simulink model "EVSimulation"  (R2020b)
settings: Solver=VariableStepAuto  StartTime=0.0  StopTime=600  FixedStep=0.5  RelTol=1e-3
model workspace (MAT data in the model file):
  AccessoryLoad = 0
  Af = 1.8
  C0 = 0.02
  Cd = 0.48
  airDensity = 1.225
  beta = 0
  energyCapacity = 30
  g = 9.81
  gearboxEfficiency = 90
  internalResistance = 0.05
  m = 840
  maxBrakeForce = 2000
  motorEfficiency = 90
  motorMaxPower = 40000
  motorMaxTorque = 83
  openCircuitVoltage = 140
  regenFraction = 1
  wheelRadius = 0.29
  windVel = 0
libraries: simulink x2, autolibshared x1, pid_lib x1
settings Model: SimulationMode=accelerator  OrderedModelArguments=off  Creator=Caleb  LastModifiedBy=Caleb

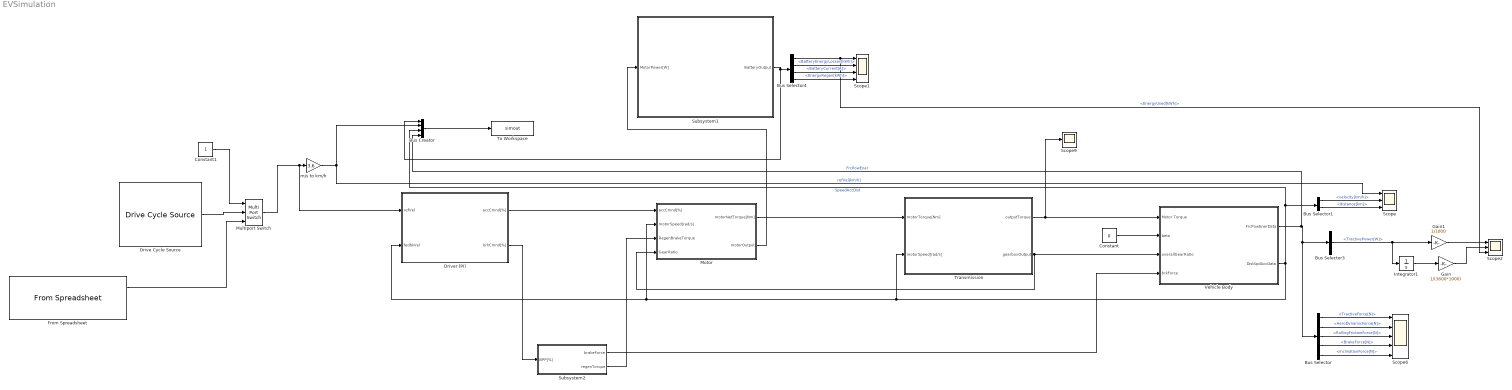
== system EVSimulation ==
  Bus Creator : BusCreator  Inputs=4
  Bus Selector : BusSelector  OutputSignals=TractiveForce[N],AeroDynamicForce[N],RollingFrictionForce[N],BrakeForce[N],InclinationForce[N]
  Bus Selector1 : BusSelector  OutputSignals=velocity[km/h],distance[km]
  Bus Selector3 : BusSelector  OutputSignals=TractivePower[W]
  Bus Selector4 : BusSelector  OutputSignals=EnergyUsed[kWh],BatteryEnergyLosses[kWh],BatteryCurrent[A],EnergyRegen[kWh]
  Constant : Constant  Value=0
  Constant1 : Constant
  Drive Cycle Source : autolibshared/Drive Cycle Source  cycleVar=US06  fileVar=cycleFTP75.mat  tfinal="600  seconds, Cyclic"  cycleRepeat=on  outAccPort=off  outGearPort=off  gearList=No gear data  t_wot1=5  xdot_woto=0  xdot_wot1=30  t_wot2=20  xdot_wot2=0  t_wotend=30  srcUnit=m/s  outUnit=m/s  srcAccUnit=m/s/s  outAccUnit=m/s^2  dt=0  aMode=1  faultOption=off  velBnd=2  velBndUnit=mph  inUnit=m/s  timeBnd=1  failOption=off  stopSim=off  maxFaultCnt=10  maxFaultTime=2  maxTotFaultTime=15  traceOption=off  dtTrace=1  traceWindow=10  lastDCname=FTP75 Velocity  lastOutUnit=mph  lastDT=0  lastTB=1  lastSB=2  forceCalcBound=off
      settings: SourceProductBaseCode=PW,MT,UV,VE,VP
  Driver (PI) : Subsystem
  From Spreadsheet : FromSpreadsheet  FileName=SpeedInputDrivecyle.xlsx  SheetName=Sheet2  ExtrapolationAfterLastDataPoint=Hold last value
  Gain : Gain  Gain=1/(3600*1000)
  Gain1 : Gain  Gain=1/1000
  Integrator1 : Integrator
  Motor : Subsystem
  Multiport Switch : MultiPortSwitch  Inputs=2
  Scope : Scope  NumInputPorts=3
  Scope1 : Scope  NumInputPorts=4
  Scope2 : Scope  NumInputPorts=3
  Scope6 : Scope  NumInputPorts=5
  Scope9 : Scope
  Subsystem1 : Subsystem
  Subsystem2 : Subsystem
  To Workspace : ToWorkspace  VariableName=simout  SaveFormat=Timeseries  SampleTime=-1
  Transmission : Subsystem
  Vehicle Body : Subsystem
  m/s to km/h : Gain  Gain=3.6
  wires:
  Motor/1(motorNetTorque[Nm]) -> Transmission/1(motorTorque[Nm])
  Transmission/1(outputTorque) -> Scope9/1, Vehicle Body/1(Motor Torque)
  Transmission/2(gearboxOutput) -> Motor/4(GearRatio), Vehicle Body/3(overallGearRatio)
  m/s to km/h/1 -> Bus Creator/2, Scope/1  "refVel[km/h]"
  Vehicle Body/1(FrcPowEnerData) -> Bus Creator/4, Bus Selector/1, Bus Selector3/1  "FrcPowEner"
  Vehicle Body/2(DistSpdAccData) -> Transmission/2(motorSpeed[rad/s]), Motor/2(motorSpeed[rad/s]), Driver (PI)/2(fedbkVel), Bus Creator/3, Bus Selector1/1  "SpeedAccDist"
  Bus Selector1/1 -> Scope/2  "<velocity[km/h]>"
  Bus Selector/5 -> Scope6/5  "<InclinationForce[N]>"
  Bus Selector3/1 -> Integrator1/1, Gain1/1  "<TractivePower[W]>"
  Subsystem1/1(BatteryOutput) -> Bus Creator/1, Bus Selector4/1
  Bus Selector4/1 -> Scope2/3, Scope1/1  "<EnergyUsed[kWh]>"
  Drive Cycle Source/1 -> Multiport Switch/2
  Bus Selector1/2 -> Scope/3  "<distance[km]>"
  Multiport Switch/1 -> Driver (PI)/1(refVel), m/s to km/h/1
  From Spreadsheet/1 -> Multiport Switch/3
  Constant1/1 -> Multiport Switch/1
  Integrator1/1 -> Gain/1
  Gain/1 -> Scope2/2
  Motor/2(motorOutput) -> Subsystem1/1(MotorPower[W])
  Bus Selector4/2 -> Scope1/2  "<BatteryEnergyLosses[kWh]>"
  Bus Selector4/3 -> Scope1/3  "<BatteryCurrent[A]>"
  Bus Creator/1 -> To Workspace/1
  Bus Selector/1 -> Scope6/1  "<TractiveForce[N]>"
  Driver (PI)/1(accCmnd[%]) -> Motor/1(accCmnd[%])
  Driver (PI)/2(brkCmnd[%]) -> Subsystem2/1(BPP[%])
  Gain1/1 -> Scope2/1
  Bus Selector/2 -> Scope6/2  "<AeroDynamicForce[N]>"
  Bus Selector/3 -> Scope6/3  "<RollingFrictionForce[N]>"
  Bus Selector/4 -> Scope6/4  "<BrakeForce[N]>"
  Constant/1 -> Vehicle Body/2(beta)
  Subsystem2/1(brakeForce) -> Vehicle Body/4(brkForce)
  Subsystem2/2(regenTorque) -> Motor/3(RegenBrakeTorque)
  Bus Selector4/4 -> Scope1/4  "<EnergyRegen[kWh]>"

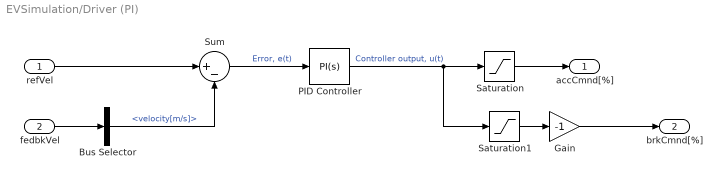
== system EVSimulation/Driver (PI) ==
  refVel : Inport
  fedbkVel : Inport  Port=2
  Bus Selector : BusSelector  OutputSignals=velocity[m/s]
  Gain : Gain  Gain=-1
  PID Controller : pid_lib/PID Controller  Controller=PI  Form=Parallel  TimeDomain=Continuous-time  UseExternalTs=off  SampleTime=-1  IntegratorMethod=Forward Euler  FilterMethod=Forward Euler  ControllerParametersSource=internal  P=200  I=1  D=0  UseFilter=on  N=1  TunerSelectOption=Transfer Function Based (PID Tuner App)  InitialConditionSource=internal  InitialConditionForIntegrator=0  InitialConditionForFilter=0  DifferentiatorICPrevScaledInput=0  ExternalReset=none  TrackingMode=off  Kt=1  LimitOutput=off  SatLimitsSource=internal  UpperSaturationLimit=inf  LowerSaturationLimit=-inf  LinearizeAsGain=on  AntiWindupMode=clamping  Kb=1  POutMin=[]  POutMax=[]  IOutMin=[]  IOutMax=[]  DOutMin=[]  DOutMax=[]  NOutMin=[]  NOutMax=[]  SumOutMin=[]  SumOutMax=[]  SaturationOutMin=[]  SaturationOutMax=[]  PParamMin=[]  PParamMax=[]  IParamMin=[]  IParamMax=[]  DParamMin=[]  DParamMax=[]  NParamMin=[]  NParamMax=[]  KbParamMin=[]  KbParamMax=[]  KtParamMin=[]  KtParamMax=[]  KbOutMin=[]  KbOutMax=[]  KtOutMin=[]  KtOutMax=[]  IntegratorOutMin=[]  IntegratorOutMax=[]  FilterOutMin=[]  FilterOutMax=[]  SumI1OutMin=[]  SumI1OutMax=[]  SumI2OutMin=[]  SumI2OutMax=[]  SumI3OutMin=[]  SumI3OutMax=[]  SumI4OutMin=[]  SumI4OutMax=[]  SumDOutMin=[]  SumDOutMax=[]  DifferentiatorOutMin=[]  DifferentiatorOutMax=[]  FilterDiffOutCoefMin=[]  FilterDiffOutCoefMax=[]  ReciprocalOutMin=[]  ReciprocalOutMax=[]  SumDenOutMin=[]  SumDenOutMax=[]  SumNumOutMin=[]  SumNumOutMax=[]  DivideOutMin=[]  DivideOutMax=[]  UdiffTsProdOutMin=[]  UdiffTsProdOutMax=[]  NTsProdOutMin=[]  NTsProdOutMax=[]  UintegralTsProdOutMin=[]  UintegralTsProdOutMax=[]  UngainTsProdOutMin=[]  UngainTsProdOutMax=[]  IntegratorContinuousStateAttributes=''  IntegratorStateMustResolveToSignalObject=off  IntegratorRTWStateStorageClass=Auto  FilterContinuousStateAttributes=''  FilterStateMustResolveToSignalObject=off  FilterRTWStateStorageClass=Auto  ParallelPVariant=InternalParameters  IdealPVariant=Disabled  IVariant=InternalParameters  DVariant=Disabled  IntegratorVariant=Continuous  SatVariant=Disabled  AWVariant=Passthrough  PCopyVariant=Disabled  TRVariant=Disabled  FdbkBlocksVariant=Forward  IdealPFdbkVariant=Disabled  SatFdbkVariant=Disabled  DerivativeFilterVariant=Disabled  NVariant=Disabled  NCopyVariant=Disabled_SignalSpec  FilterICVariant=Disabled  IntegratorICVariant=InternalICs  ExternalResetVariant=Disabled  TRSumVariant=Passthrough  SumFdbkVariant=Disabled  SumVariant=Sum_PI  TsampFilterVariant=InternalTs  TsampNgainVariant=Passthrough  TsampIntegralVariant=Passthrough  ExternalSaturationOutDataTypeStr=Inherit: Same as second input
  Saturation : Saturate  UpperLimit=100  LowerLimit=0
  Saturation1 : Saturate  UpperLimit=0  LowerLimit=-100
  Sum : Sum  Inputs=|+-
  accCmnd[%] : Outport
  brkCmnd[%] : Outport  Port=2
  wires:
  PID Controller/1 -> Saturation1/1, Saturation/1  "Controller output, u(t)"
  Sum/1 -> PID Controller/1  "Error, e(t)"
  refVel/1 -> Sum/1
  Saturation/1 -> accCmnd[%]/1
  Saturation1/1 -> Gain/1
  Gain/1 -> brkCmnd[%]/1
  fedbkVel/1 -> Bus Selector/1
  Bus Selector/1 -> Sum/2  "<velocity[m/s]>"

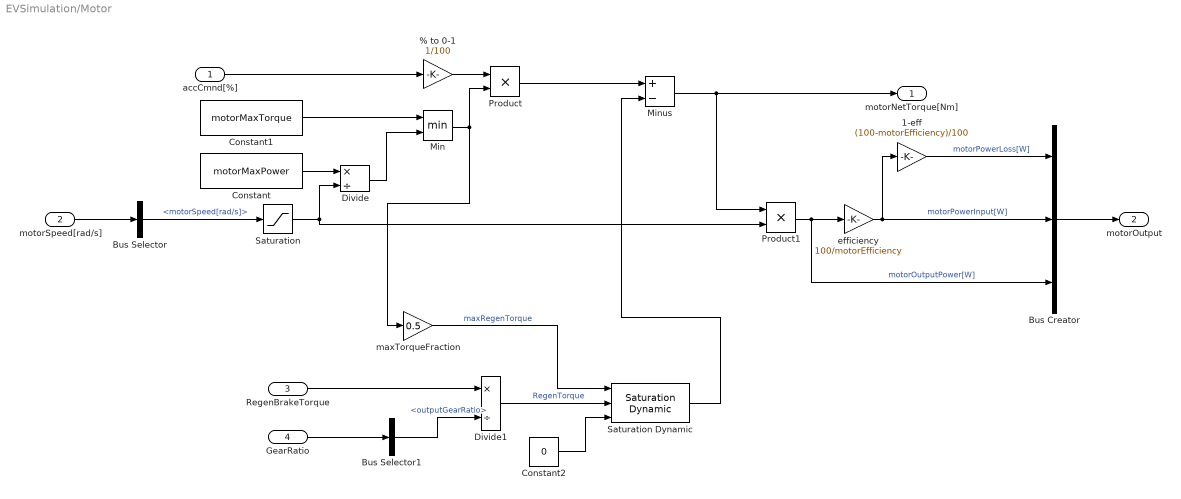
== system EVSimulation/Motor ==
  accCmnd[%] : Inport
  motorSpeed[rad/s] : Inport  Port=2
  RegenBrakeTorque : Inport  Port=3
  GearRatio : Inport  Port=4
  % to 0-1 : Gain  Gain=1/100
  1-eff : Gain  Gain=(100-motorEfficiency)/100
  Bus Creator : BusCreator  Inputs=3
  Bus Selector : BusSelector  OutputSignals=motorSpeed[rad/s]
  Bus Selector1 : BusSelector  OutputSignals=outputGearRatio
  Constant : Constant  Value=motorMaxPower
  Constant1 : Constant  Value=motorMaxTorque
  Constant2 : Constant  Value=0
  Divide : Product  Inputs=*/
  Divide1 : Product  Inputs=*/
  Min : MinMax  Inputs=2
  Minus : Sum  Inputs=+-
  Product : Product
  Product1 : Product
  Saturation : Saturate  UpperLimit=inf  LowerLimit=0.00001
  Saturation Dynamic : simulink/Discontinuities/Saturation Dynamic  OutMin=[]  OutMax=[]  OutDataTypeStr=Inherit: Same as second input  OutDataType=fixdt(1, 16)  OutScaling=2^-10  DoSatur=off
  efficiency : Gain  Gain=100/motorEfficiency
  maxTorqueFraction : Gain  Gain=0.5
  motorNetTorque[Nm] : Outport
  motorOutput : Outport  Port=2
  wires:
  accCmnd[%]/1 -> % to 0-1/1
  Constant1/1 -> Min/1
  Min/1 -> Product/2, maxTorqueFraction/1
  Divide/1 -> Min/2
  Constant/1 -> Divide/1
  Product1/1 -> Bus Creator/3, efficiency/1  "motorOutputPower[W]"
  % to 0-1/1 -> Product/1
  Saturation/1 -> Divide/2, Product1/2
  motorSpeed[rad/s]/1 -> Bus Selector/1
  Bus Selector/1 -> Saturation/1  "<motorSpeed[rad/s]>"
  Product/1 -> Minus/1
  efficiency/1 -> 1-eff/1, Bus Creator/2  "motorPowerInput[W]"
  1-eff/1 -> Bus Creator/1  "motorPowerLoss[W]"
  Bus Creator/1 -> motorOutput/1
  RegenBrakeTorque/1 -> Divide1/1
  GearRatio/1 -> Bus Selector1/1
  Divide1/1 -> Saturation Dynamic/2  "RegenTorque"
  maxTorqueFraction/1 -> Saturation Dynamic/1  "maxRegenTorque"
  Constant2/1 -> Saturation Dynamic/3
  Minus/1 -> Product1/1, motorNetTorque[Nm]/1
  Saturation Dynamic/1 -> Minus/2
  Bus Selector1/1 -> Divide1/2  "<outputGearRatio>"

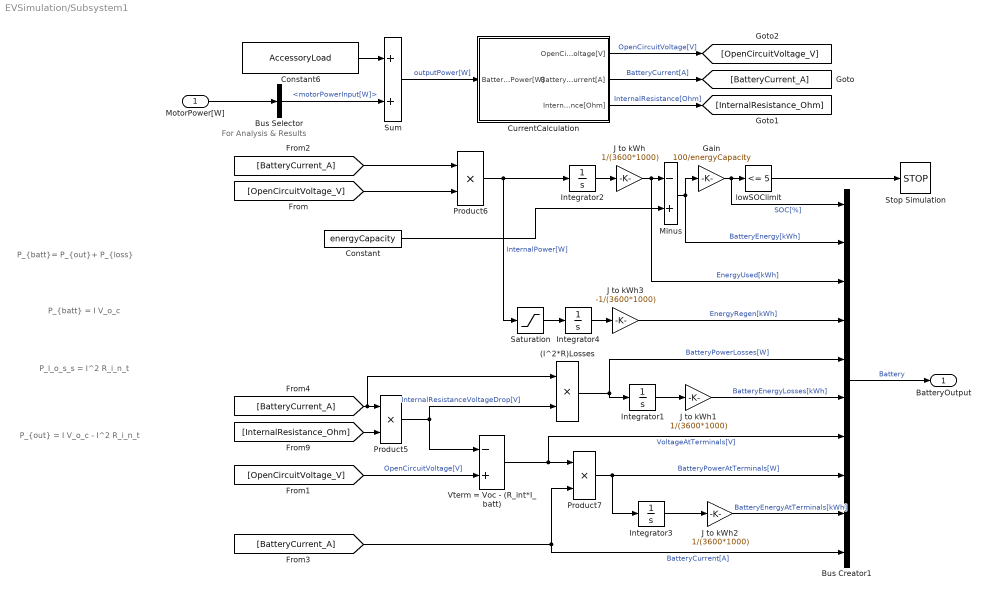
== system EVSimulation/Subsystem1 ==
  note: P_{batt}= P_{out}+ P_{loss}
  note: For Analysis & Results
  note: P_{out} = I V_o_c - I^2 R_i_n_t
  note: P_{batt} = I V_o_c
  note: P_l_o_s_s = I^2 R_i_n_t
  MotorPower[W] : Inport
  (I^2*R)Losses : Product  RndMeth=Zero
  Bus Creator1 : BusCreator  Inputs=10
  Bus Selector : BusSelector  OutputSignals=motorPowerInput[W]
  Constant : Constant  Value=energyCapacity
  Constant6 : Constant  Value=AccessoryLoad
  CurrentCalculation : Subsystem
  Gain : Gain  Gain=100/energyCapacity
  Integrator1 : Integrator  ZeroCross=off
  Integrator2 : Integrator  ZeroCross=off
  Integrator3 : Integrator
  Integrator4 : Integrator  ZeroCross=off
  J to kWh : Gain  Gain=1/(3600*1000)
  J to kWh1 : Gain  Gain=1/(3600*1000)
  J to kWh2 : Gain  Gain=1/(3600*1000)
  J to kWh3 : Gain  Gain=-1/(3600*1000)
  Minus : Sum  Inputs=-+
  Product5 : Product  RndMeth=Zero
  Product6 : Product  RndMeth=Zero
  Product7 : Product  RndMeth=Zero
  Saturation : Saturate  UpperLimit=0  LowerLimit=-inf
  Stop Simulation : Stop
  Sum : Sum
  Vterm = Voc - (R_int*I_batt) : Sum  Inputs=-+
  lowSOClimit : simulink/Logic and Bit Operations/Compare To Constant  relop=<=  const=5  OutDataTypeStr=boolean
  BatteryOutput : Outport  VectorParamsAs1DForOutWhenUnconnected=off
  wires:
  Product7/1 -> Bus Creator1/8, Integrator3/1  "BatteryPowerAtTerminals[W]"
  [BatteryCurrent_A] -> Product7/2, Bus Creator1/10  "BatteryCurrent[A]"
  CurrentCalculation/1(OpenCircuitVoltage[V]) -> [OpenCircuitVoltage_V]  "OpenCircuitVoltage[V]"
  Gain/1 -> Bus Creator1/1, lowSOClimit/1  "SOC[%]"
  lowSOClimit/1 -> Stop Simulation/1
  MotorPower[W]/1 -> Bus Selector/1
  [BatteryCurrent_A] -> Product6/1
  [InternalResistance_Ohm] -> Product5/2
  Product5/1 -> (I^2*R)Losses/2, Vterm = Voc - (R_int*I_batt)/1  "InternalResistanceVoltageDrop[V]"
  Sum/1 -> CurrentCalculation/1(BatteryPower[W])  "outputPower[W]"
  Vterm = Voc - (R_int*I_batt)/1 -> Bus Creator1/7, Product7/1  "VoltageAtTerminals[V]"
  [OpenCircuitVoltage_V] -> Vterm = Voc - (R_int*I_batt)/2  "OpenCircuitVoltage[V]"
  (I^2*R)Losses/1 -> Bus Creator1/5, Integrator1/1  "BatteryPowerLosses[W]"
  [OpenCircuitVoltage_V] -> Product6/2
  Integrator2/1 -> J to kWh/1
  Integrator1/1 -> J to kWh1/1
  Constant6/1 -> Sum/1
  [BatteryCurrent_A] -> (I^2*R)Losses/1, Product5/1
  Integrator3/1 -> J to kWh2/1
  Product6/1 -> Integrator2/1, Saturation/1  "InternalPower[W]"
  CurrentCalculation/2(BatteryCurrent[A]) -> [BatteryCurrent_A]  "BatteryCurrent[A]"
  CurrentCalculation/3(InternalResistance[Ohm]) -> [InternalResistance_Ohm]  "InternalResistance[Ohm]"
  Bus Creator1/1 -> BatteryOutput/1  "Battery"
  Bus Selector/1 -> Sum/2  "<motorPowerInput[W]>"
  J to kWh/1 -> Bus Creator1/3, Minus/1  "EnergyUsed[kWh]"
  Constant/1 -> Minus/2
  Minus/1 -> Bus Creator1/2, Gain/1  "BatteryEnergy[kWh]"
  J to kWh1/1 -> Bus Creator1/6  "BatteryEnergyLosses[kWh]"
  J to kWh2/1 -> Bus Creator1/9  "BatteryEnergyAtTerminals[kWh]"
  Saturation/1 -> Integrator4/1
  Integrator4/1 -> J to kWh3/1
  J to kWh3/1 -> Bus Creator1/4  "EnergyRegen[kWh]"

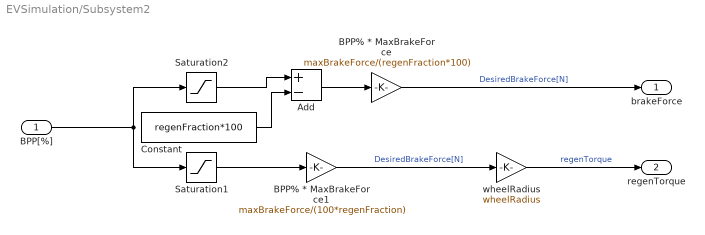
== system EVSimulation/Subsystem2 ==
  BPP[%] : Inport
  Add : Sum  Inputs=+-
  BPP% * MaxBrakeForce : Gain  Gain=maxBrakeForce/(regenFraction*100)
  BPP% * MaxBrakeForce1 : Gain  Gain=maxBrakeForce/(100*regenFraction)
  Constant : Constant  Value=regenFraction*100
  Saturation1 : Saturate  UpperLimit=regenFraction*100  LowerLimit=0
  Saturation2 : Saturate  UpperLimit=100  LowerLimit=regenFraction*100
  wheelRadius : Gain  Gain=wheelRadius
  brakeForce : Outport
  regenTorque : Outport  Port=2
  wires:
  wheelRadius/1 -> regenTorque/1  "regenTorque"
  BPP[%]/1 -> Saturation1/1, Saturation2/1
  BPP% * MaxBrakeForce1/1 -> wheelRadius/1  "DesiredBrakeForce[N]"
  Saturation1/1 -> BPP% * MaxBrakeForce1/1
  BPP% * MaxBrakeForce/1 -> brakeForce/1  "DesiredBrakeForce[N]"
  Saturation2/1 -> Add/1
  Constant/1 -> Add/2
  Add/1 -> BPP% * MaxBrakeForce/1

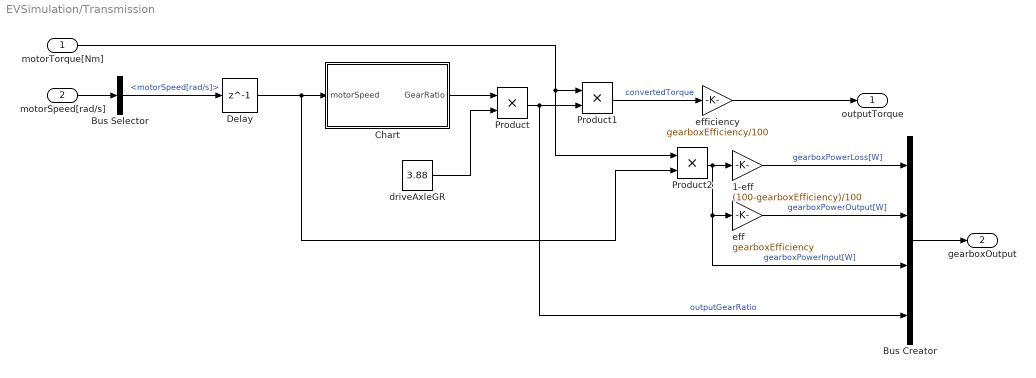
== system EVSimulation/Transmission ==
  motorTorque[Nm] : Inport
  motorSpeed[rad/s] : Inport  Port=2
  1-eff : Gain  Gain=(100-gearboxEfficiency)/100
  Bus Creator : BusCreator  Inputs=4
  Bus Selector : BusSelector  OutputSignals=motorSpeed[rad/s]
  Chart : Stateflow chart  TreatAsAtomicUnit=on
  Delay : Delay  DelayLength=1  InitialCondition=0.0001
  Product : Product
  Product1 : Product
  Product2 : Product
  driveAxleGR : Constant  Value=3.88
  eff : Gain  Gain=gearboxEfficiency
  efficiency : Gain  Gain=gearboxEfficiency/100
  outputTorque : Outport
  gearboxOutput : Outport  Port=2
  wires:
  Product/1 -> Bus Creator/4, Product1/2  "outputGearRatio"
  driveAxleGR/1 -> Product/2
  Product1/1 -> efficiency/1  "convertedTorque"
  Chart/1(GearRatio) -> Product/1
  motorTorque[Nm]/1 -> Product1/1, Product2/1
  motorSpeed[rad/s]/1 -> Bus Selector/1
  Delay/1 -> Chart/1(motorSpeed), Product2/2
  Bus Selector/1 -> Delay/1  "<motorSpeed[rad/s]>"
  efficiency/1 -> outputTorque/1
  Product2/1 -> 1-eff/1, Bus Creator/3, eff/1  "gearboxPowerInput[W]"
  1-eff/1 -> Bus Creator/1  "gearboxPowerLoss[W]"
  eff/1 -> Bus Creator/2  "gearboxPowerOutput[W]"
  Bus Creator/1 -> gearboxOutput/1

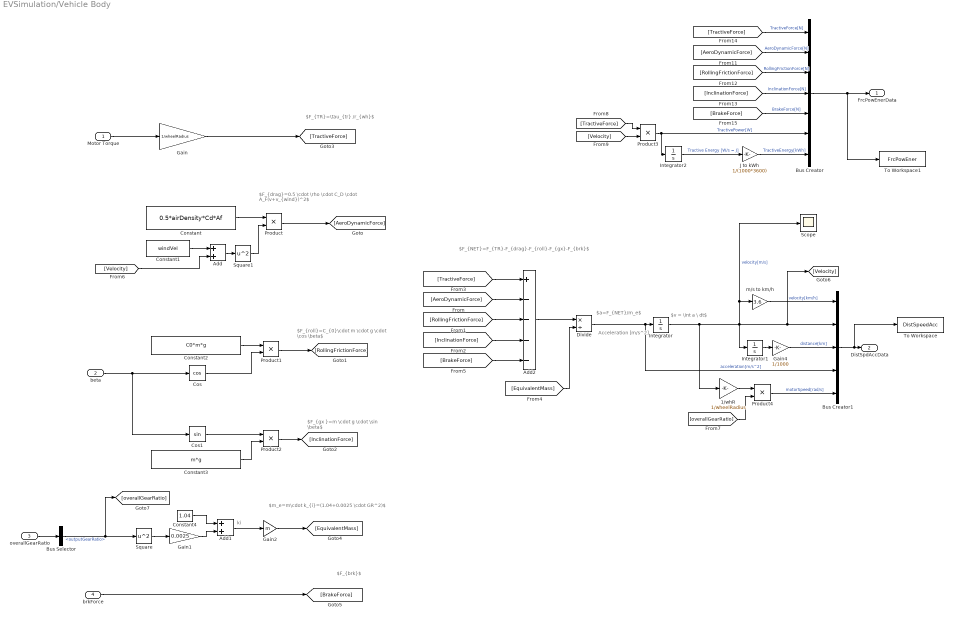
== system EVSimulation/Vehicle Body ==
  note: $v = \int a \ dt$
  note: $F_{roll}=C_{0}\cdot m \cdot g \cdot \cos \beta$
  note: Acceleration [m/s^2]
  note: ki
  note: $F_{gx }=m \cdot g \cdot \sin \beta$
  note: $F_{drag}=0.5 \cdot \rho \cdot C_D \cdot A_F(v+v_{wind})^2$
  note: $F_{TR}=\tau_{tr} /r_{wh}$
  note: $m_e=m\cdot k_{i}=(1.04+0.0025 \cdot GR^2)$
  note: $F_{brk}$
  note: $F_{NET}=F_{TR}-F_{drag}-F_{roll}-F_{gx}-F_{brk}$
  note: $a=F_{NET}/m_e$
  Motor Torque : Inport
  beta : Inport  Port=2
  overallGearRatio : Inport  Port=3
  brkForce : Inport  Port=4
  1/whR : Gain  Gain=1/wheelRadius
  Add : Sum
  Add1 : Sum
  Add2 : Sum  Inputs=+----
  Bus Creator : BusCreator  Inputs=7
  Bus Creator1 : BusCreator  Inputs=5
  Bus Selector : BusSelector  OutputSignals=outputGearRatio
  Constant : Constant  Value=0.5*airDensity*Cd*Af
  Constant1 : Constant  Value=windVel
  Constant2 : Constant  Value=C0*m*g
  Constant3 : Constant  Value=m*g
  Constant4 : Constant  Value=1.04
  Cos : Trigonometry  Operator=cos
  Cos1 : Trigonometry
  Divide : Product  Inputs=*/
  Gain : Gain  Gain=1/wheelRadius
  Gain1 : Gain  Gain=0.0025
  Gain2 : Gain  Gain=m
  Gain4 : Gain  Gain=1/1000
  Integrator : Integrator
  Integrator1 : Integrator
  Integrator2 : Integrator
  J to kWh : Gain  Gain=1/(1000*3600)
  Product{,1..4} (5 alike) : Product
  Scope : Scope
  Square : Math  Operator=square  SaturateOnIntegerOverflow=on
  Square1 : Math  Operator=square  SaturateOnIntegerOverflow=on
  To Workspace : ToWorkspace  VariableName=DistSpeedAcc  SaveFormat=Timeseries  SampleTime=-1
  To Workspace1 : ToWorkspace  VariableName=FrcPowEner  SaveFormat=Timeseries  SampleTime=-1
  m/s to km/h : Gain  Gain=3.6
  FrcPowEnerData : Outport
  DistSpdAccData : Outport  Port=2
  wires:
  Motor Torque/1 -> Gain/1
  Constant/1 -> Product/1
  Square/1 -> Gain1/1
  Product1/1 -> [RollingFrictionForce]
  overallGearRatio/1 -> Bus Selector/1
  [RollingFrictionForce] -> Add2/3
  [AeroDynamicForce] -> Add2/2
  Product/1 -> [AeroDynamicForce]
  Gain/1 -> [TractiveForce]
  Product2/1 -> [InclinationForce]
  [EquivalentMass] -> Divide/2
  Gain1/1 -> Add1/2
  Constant1/1 -> Add/1
  Integrator/1 -> m/s to km/h/1, Scope/1, Bus Creator1/2, [Velocity], Integrator1/1, 1/whR/1  "velocity[m/s]"
  beta/1 -> Cos1/1, Cos/1
  [InclinationForce] -> Add2/4
  [TractiveForce] -> Add2/1
  Add1/1 -> Gain2/1
  Constant2/1 -> Product1/1
  Constant4/1 -> Add1/1
  Constant3/1 -> Product2/2
  Cos1/1 -> Product2/1
  Cos/1 -> Product1/2
  Gain2/1 -> [EquivalentMass]
  Add2/1 -> Divide/1
  Divide/1 -> Bus Creator1/4, Integrator/1  "acceleration[m/s^2]"
  1/whR/1 -> Product4/1
  Product4/1 -> Bus Creator1/5  "motorSpeed[rad/s]"
  [BrakeForce] -> Add2/5
  brkForce/1 -> [BrakeForce]
  [overallGearRatio] -> Product4/2
  [TractiveForce] -> Product3/1
  [Velocity] -> Product3/2
  m/s to km/h/1 -> Bus Creator1/1  "velocity[km/h]"
  [TractiveForce] -> Bus Creator/1  "TractiveForce[N]"
  [AeroDynamicForce] -> Bus Creator/2  "AeroDynamicForce[N]"
  [RollingFrictionForce] -> Bus Creator/3  "RollingFrictionForce[N]"
  [InclinationForce] -> Bus Creator/4  "InclinationForce[N]"
  [BrakeForce] -> Bus Creator/5  "BrakeForce[N]"
  Product3/1 -> Bus Creator/6, Integrator2/1  "TractivePower[W]"
  Bus Creator/1 -> FrcPowEnerData/1, To Workspace1/1
  Add/1 -> Square1/1
  Square1/1 -> Product/2
  Integrator1/1 -> Gain4/1
  Gain4/1 -> Bus Creator1/3  "distance[km]"
  Bus Creator1/1 -> To Workspace/1, DistSpdAccData/1
  Integrator2/1 -> J to kWh/1  "Tractive Energy [W/s = J]"
  J to kWh/1 -> Bus Creator/7  "TractiveEnergy[kWh]"
  [Velocity] -> Add/2
  Bus Selector/1 -> [overallGearRatio], Square/1  "<outputGearRatio>"

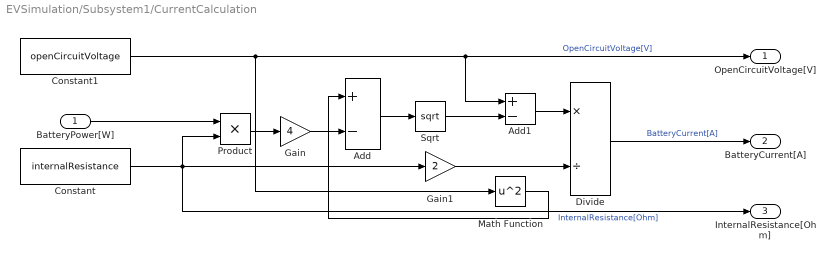
== system EVSimulation/Subsystem1/CurrentCalculation ==
  BatteryPower[W] : Inport
  Add : Sum  Inputs=+-
  Add1 : Sum  Inputs=+-
  Constant : Constant  Value=internalResistance
  Constant1 : Constant  Value=openCircuitVoltage
  Divide : Product  Inputs=*/
  Gain : Gain  Gain=4
  Gain1 : Gain  Gain=2
  Math Function : Math  Operator=square  SignedPower=on  SaturateOnIntegerOverflow=on
  Product : Product  RndMeth=Zero
  Sqrt : Sqrt  SaturateOnIntegerOverflow=on
  OpenCircuitVoltage[V] : Outport  VectorParamsAs1DForOutWhenUnconnected=off
  BatteryCurrent[A] : Outport  Port=2  VectorParamsAs1DForOutWhenUnconnected=off
  InternalResistance[Ohm] : Outport  Port=3  VectorParamsAs1DForOutWhenUnconnected=off
  wires:
  BatteryPower[W]/1 -> Product/1
  Constant/1 -> InternalResistance[Ohm]/1, Gain1/1, Product/2  "InternalResistance[Ohm]"
  Product/1 -> Gain/1
  Constant1/1 -> Math Function/1, OpenCircuitVoltage[V]/1, Add1/1  "OpenCircuitVoltage[V]"
  Math Function/1 -> Add/1
  Gain/1 -> Add/2
  Sqrt/1 -> Add1/2
  Add/1 -> Sqrt/1
  Add1/1 -> Divide/1
  Gain1/1 -> Divide/2
  Divide/1 -> BatteryCurrent[A]/1  "BatteryCurrent[A]"

== stateflow chart EVSimulation/Transmission/Chart ==
  state FIRST
    entry:
    GearRatio=3.116;
  state SECOND
    entry:
    GearRatio=1.882;
  state THIRD
    entry:
    GearRatio=1.296;
  state FOURTH
    entry:
    GearRatio=0.972;
  state FIFTH
    entry:
    GearRatio=0.738;
  (default) -> FIRST
  SECOND -> FIRST [order 1] : [motorSpeed<350]
  FIRST -> SECOND : [motorSpeed>750]
  THIRD -> SECOND [order 1] : [motorSpeed<400]
  SECOND -> THIRD [order 2] : [motorSpeed>700]
  FOURTH -> THIRD [order 1] : [motorSpeed<400]
  THIRD -> FOURTH [order 2] : [motorSpeed>700]
  FIFTH -> FOURTH : [motorSpeed<400]
  FOURTH -> FIFTH [order 2] : [motorSpeed>700]
  data: motorSpeed input; GearRatio output
